simulink model "RadarSimulinkProjectRev001b"  (R2024a)
settings: Solver=VariableStepAuto  StartTime=0.0  StopTime=0.001  RelTol=1e-3
values from neighbouring files (symbols this model uses):
  AngleTime = SweepTime/10    (= 10000)    [InitializationOfVariables.m]    (also in InitializationOfVariablesRev000.m; InitializationOfVariablesRev001.m; InitializationOfVariablesRev003.m = 2097152; InitializationOfVariablesRev004.m = 2097152)
  Btn_Debounce = 20000    [InitializationOfVariablesRev003.m]    (also in InitializationOfVariablesRev004.m)
  FreqDeltaPeriod = 45    [InitializationOfVariablesRev003.m]    (also in InitializationOfVariablesRev004.m = 1)
  RXFFTLength = 16384    [InitializationOfVariablesRev003.m]    (also in InitializationOfVariablesRev004.m = 2048)
  SweepTime = 100000    [InitializationOfVariables.m]    (also in InitializationOfVariablesRev000.m; InitializationOfVariablesRev001.m; InitializationOfVariablesRev003.m = 23068672; InitializationOfVariablesRev004.m = 23068672)
undefined symbols (not defined in the file or in its folder): SignalGenerationForAnalysis, Subsystem, xc7a200tfbg676
libraries: hdlBasic x75, hdlDSPIP x6, hdlUtilities x1, vmcUtilities x1
settings Model: Creator=Cube II  LastModifiedBy=Cube II

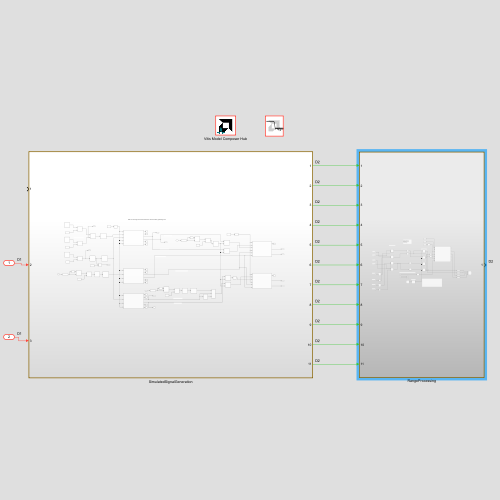
[thumbnail: Simulink's stored preview of the top-level diagram]
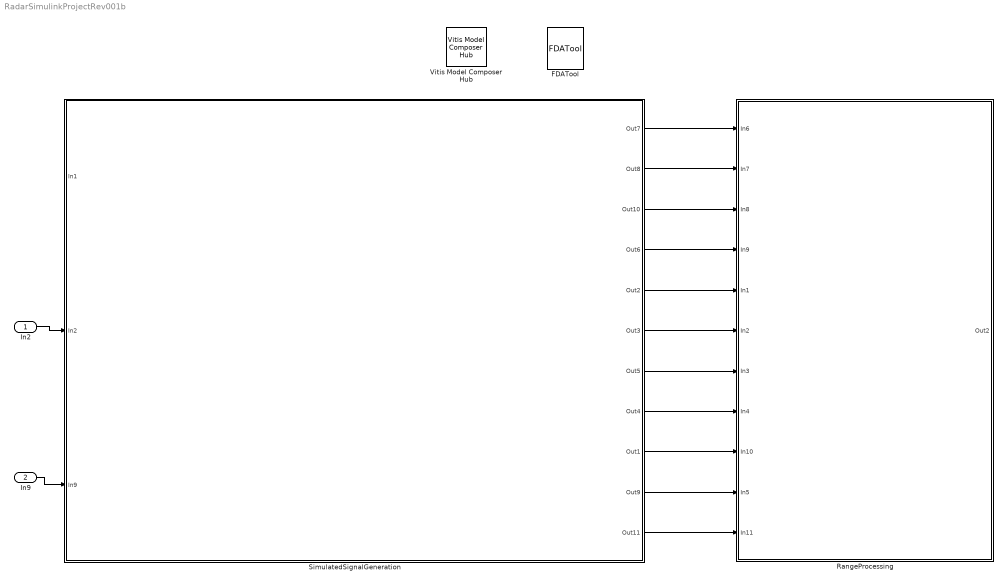
== system RadarSimulinkProjectRev001b ==
  In2 : Inport
  In9 : Inport  Port=2
  FDATool : hdlUtilities/FDATool  block_type=fdatool
      settings: infoedit=FDATool
  RangeProcessing : Subsystem
  SimulatedSignalGeneration : Subsystem  SystemSampleTime=1/200e6
  Vitis Model Composer Hub : vmcUtilities/Vitis Model Composer Hub  Tag=genX  CodeGeneration=off  SubsystemName=Subsystem  BlockHierPath=SignalGenerationForAnalysis/Subsystem  CompilationType=HDLCompilation  SubsystemType=HDLNode  ExportTypeV2=IP Catalog  StartColumn=1  NumberOfColumns=1  TargetDirectory=./netlist  exportDesign=off  analyzeDesign=on  validateDesignOnHw=off  ExportType=AI Engines  IpVendor=xilinx.com  IpLibrary=hls  IpVersion=1.0  IpHWLanguage=Verilog  AieCompilerOptions={}  AieSimulatorOptions={}  CreateTestbench=on  TestbenchStackSize=10  RunRtlSim=off  RunCSim=off  RunAieSim=off  AieSimTimeout=50000  RunAieSimProfiling=off  LaunchVitisAnalyzer=off  PlotOutput=off  RunX86Sim=off  X86SimTimeout=10  GenHwImage=off  GenLibadfXo=on  GenHwValidationCode=off  PlatformType=Not Specified  HwSystemType=Baremetal  HwValidationTarget=hw  ProjDevice=Artix-7 AC701 Evaluation Platform (xc7a200tfbg676-2)  ProjDevicePart=xc7a200tfbg676-2  AIEType=None  SamplePeriod=-1  ClockFrequency=200  DataPathParallelism=1  xilinxfamily=artix7  part=xc7a200t  speed=-2  package=fbg676  directory=./netlist\ip\Subsystem\src  testbench=off  incr_netlist=off  synthesis_tool=Vivado  clock_wrapper=Clock Enables  dbl_ovrd=According to Block Masks  dcm_input_clock_period=10  sysclk_period=5  simulink_period=1/200e6  eval_field=0  IPInfoJsonString="{\"DUTSubsystemName\":\"Subsystem\",\"HDLSubsystem\":{\"SubsystemName\":\"Subsystem\",\"IPName\":\"Subsystem\",\"IPLibrary\":\"VMC\",\"IPVendor\":\"User Company\",\"IPVersion\":\"1.0\",\"TargetDirectory\":\"./netlist\",\"SubsystemDir\":\"./netlist\\\\ip\\\\Subsystem\",\"FreqHz\":\"200000000\"},\"SubsystemTag\":\"HDLNode\"}"  LogFileName=S:\RadarProjectSimulink\netlist\model_composer.log  NThreads=4  IPConfigFile=C:\Users\Cube II\AppData\Local\Temp\vmctmp-5941030035629153029\SignalGenerationForAnalysis_ipconfig.json
  wires:
  In2/1 -> SimulatedSignalGeneration/2(In2)
  In9/1 -> SimulatedSignalGeneration/3(In9)
  SimulatedSignalGeneration/3(Out10) -> RangeProcessing/3(In8)
  SimulatedSignalGeneration/4(Out6) -> RangeProcessing/4(In9)
  SimulatedSignalGeneration/7(Out5) -> RangeProcessing/7(In3)
  SimulatedSignalGeneration/8(Out4) -> RangeProcessing/8(In4)
  SimulatedSignalGeneration/10(Out9) -> RangeProcessing/10(In5)
  SimulatedSignalGeneration/9(Out1) -> RangeProcessing/9(In10)
  SimulatedSignalGeneration/2(Out8) -> RangeProcessing/2(In7)
  SimulatedSignalGeneration/1(Out7) -> RangeProcessing/1(In6)
  SimulatedSignalGeneration/6(Out3) -> RangeProcessing/6(In2)
  SimulatedSignalGeneration/5(Out2) -> RangeProcessing/5(In1)
  SimulatedSignalGeneration/11(Out11) -> RangeProcessing/11(In11)

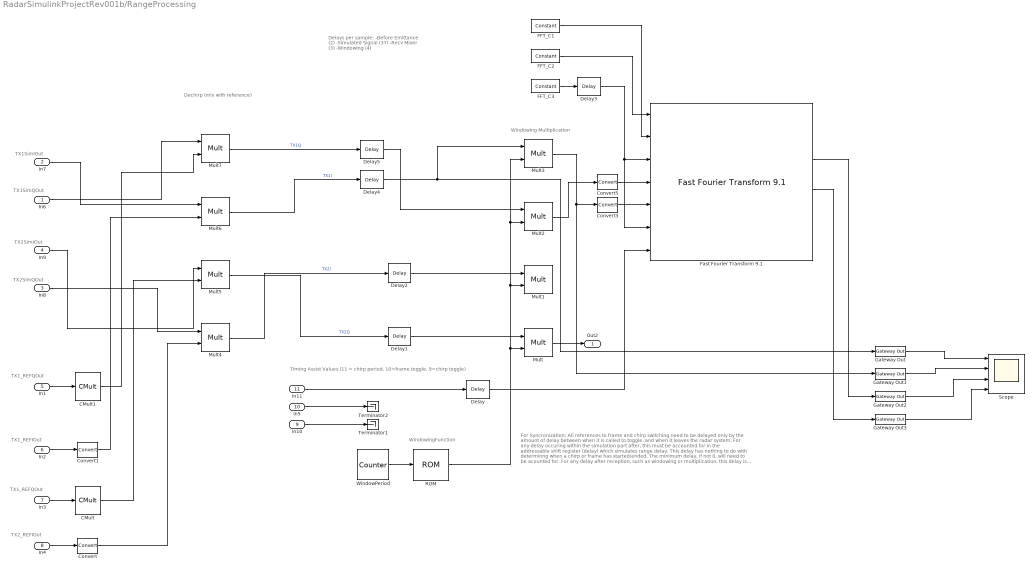
== system RadarSimulinkProjectRev001b/RangeProcessing ==
  note: Delays per sample:
      | -Before Emittance (2)
      | -Simulated Signal (37)
      | -Recv Mixer (3)
      | -Windowing (4)
  note: TX1SimIOut
  note: TX1SimQOut
  note: TX2SimIOut
  note: TX2SimQOut
  note: TX1_REFIOut
  note: TX1_REFQOut
  note: TX2_REFIOut
  note: TX1_REFQOut
  note: Dechirp (mix with reference)
  note: Timing Assist Values (11 = chirp period, 10=frame toggle, 9=chirp toggle)
  note: WindowingFunction
  note: Windowing Multiplication
  note: For Syncronization: All references to frame and chirp switching need to be delayed only by the amount of delay between when it is called to toggle, and when it leaves the radar system.
      |
      | For any delay occuring within the simulation part after, this must be accounted for in the addressable shift register (delay) which simulates range delay. This delay has nothing to do with determinng when a chirp or frame has started/ended. The minimum delay, if not 0, will need to be acounted for.
      |
      | For any delay after reception, such as windowing or multiplication, this delay is relevant to anything that has to do with the processes that depend on knowing when a frame or chirp has started/ended. Since it should only start sampling once a signal theoretically should have arrived from 0 meters (no sim delay)
  In6 : Inport
  In7 : Inport  Port=2
  In8 : Inport  Port=3
  In9 : Inport  Port=4
  In1 : Inport  Port=5
  In2 : Inport  Port=6
  In3 : Inport  Port=7
  In4 : Inport  Port=8
  In10 : Inport  Port=9
  In5 : Inport  Port=10
  In11 : Inport  Port=11
  CMult : hdlBasic/CMult  const=-1  gui_display_data_type=Fixed-point  const_n_bits=1  const_bin_pt=0  float_type=Single  exp_bits=8  fraction_bits=24  en=off  latency=0  precision=Full  arith_type="Signed  (2's comp)"  n_bits=16  bin_pt=14  quantization=Truncate  overflow=Wrap  use_behavioral_HDL=off  mem_type=Distributed RAM  pipeline=off  XmcBlockStatus=1  maskContainerNames=tabcontainer1  block_type=cmult  block_config=sysgen:CMult_config
      settings: infoedit=[]
  CMult1 : hdlBasic/CMult  const=-1  gui_display_data_type=Fixed-point  const_n_bits=1  const_bin_pt=0  float_type=Single  exp_bits=8  fraction_bits=24  en=off  latency=0  precision=Full  arith_type="Signed  (2's comp)"  n_bits=16  bin_pt=14  quantization=Truncate  overflow=Wrap  use_behavioral_HDL=off  mem_type=Distributed RAM  pipeline=off  XmcBlockStatus=1  maskContainerNames=tabcontainer1  block_type=cmult  block_config=sysgen:CMult_config
      settings: infoedit=[]
  Convert : hdlBasic/Convert  gui_display_data_type=Fixed-point  arith_type=Signed (2's comp)  n_bits=17  bin_pt=15  float_type=Single  exp_bits=8  fraction_bits=24  quantization=Truncate  overflow=Wrap  en=off  latency=0  pipeline=off  XmcBlockStatus=1  maskContainerNames=group2  block_type=convert  block_config=sysgen:Convert_config  block_width=595  block_height=885
  Convert1 : hdlBasic/Convert  gui_display_data_type=Fixed-point  arith_type=Signed (2's comp)  n_bits=17  bin_pt=15  float_type=Single  exp_bits=8  fraction_bits=24  quantization=Truncate  overflow=Wrap  en=off  latency=0  pipeline=off  XmcBlockStatus=1  maskContainerNames=group2  block_type=convert  block_config=sysgen:Convert_config  block_width=595  block_height=885
  Convert3 : hdlBasic/Convert  gui_display_data_type=Fixed-point  arith_type=Signed (2's comp)  n_bits=16  bin_pt=15  float_type=Single  exp_bits=8  fraction_bits=24  quantization=Truncate  overflow=Wrap  en=off  latency=0  pipeline=off  XmcBlockStatus=1  maskContainerNames=group2  block_type=convert  block_config=sysgen:Convert_config  block_width=595  block_height=885
  Convert5 : hdlBasic/Convert  gui_display_data_type=Fixed-point  arith_type=Signed (2's comp)  n_bits=16  bin_pt=15  float_type=Single  exp_bits=8  fraction_bits=24  quantization=Truncate  overflow=Wrap  en=off  latency=0  pipeline=off  XmcBlockStatus=1  maskContainerNames=group2  block_type=convert  block_config=sysgen:Convert_config  block_width=595  block_height=885
  Delay : hdlBasic/Delay  rst=off  en=off  latency=46  reg_retiming=off  XmcBlockStatus=1  maskContainerNames=group1  block_type=delay  block_config=sysgen:Delay_config
  Delay{1..2,4..5} (4 alike) : hdlBasic/Delay  rst=off  en=off  latency=1  reg_retiming=off  XmcBlockStatus=1  maskContainerNames=group1  block_type=delay  block_config=sysgen:Delay_config
  Delay3 : hdlBasic/Delay  rst=off  en=off  latency=46  reg_retiming=off  XmcBlockStatus=1  maskContainerNames=group1  block_type=delay  block_config=sysgen:Delay_config
  FFT_C1 : hdlBasic/Constant  const=1.0  gui_display_data_type=Fixed-point  arith_type=Unsigned  n_bits=1  bin_pt=0  preci_type=Single  exp_width=8  frac_width=24  explicit_period=on  period=1/200e6  XmcBlockStatus=1  maskContainerNames=tabcontainer1  block_type=constant  block_config=sysgen:Constant_config
  FFT_C2 : hdlBasic/Constant  const=0  gui_display_data_type=Fixed-point  arith_type=Unsigned  n_bits=12  bin_pt=0  preci_type=Single  exp_width=8  frac_width=24  explicit_period=on  period=1/200e6  XmcBlockStatus=1  maskContainerNames=tabcontainer1  block_type=constant  block_config=sysgen:Constant_config
  FFT_C3 : hdlBasic/Constant  const=1  gui_display_data_type=Boolean  arith_type=Boolean  n_bits=12  bin_pt=0  preci_type=Single  exp_width=8  frac_width=24  explicit_period=on  period=1/200e6  XmcBlockStatus=1  maskContainerNames=tabcontainer1  block_type=constant  block_config=sysgen:Constant_config
  Fast Fourier Transform 9.1 : hdlDSPIP/Fast Fourier Transform 9.1   transform_length=4096  target_clock_frequency=200  target_data_throughput=50  implementation_options=pipelined_streaming_io  run_time_configurable_transform_length=off  enable_ssr=off  super_sample_rates=1  data_format=fixed_point  phase_factor_width=24  scaling_options=scaled  rounding_modes=truncation  aclken=off  aresetn=off  output_ordering=bit_reversed_order  cyclic_prefix_insertion=off  throttle_scheme=realtime  xk_index=off  ovflo=off  trim_axipin_name=on  memory_options_data=block_ram  memory_options_phase_factors=block_ram  number_of_stages_using_block_ram_for_data_and_phase_factors=4  memory_options_reorder=block_ram  memory_options_hybrid=off  complex_mult_type=use_mults_resources  butterfly_type=use_luts  simulation_type=hybrid_sim  simulation_model=sysgen:xfftv9_cmodel  data_path_portlist={ 's_axis_data_tdata', 'm_axis_data_tdata', 'm_axis_status_tdata', 'event_fft_overflow' }  channels=1  input_ordering=natural_order  input_width=16  ip_name=Fast Fourier Transform  ip_version=9.1  dsptool_ready=true  ipcore_usecache=true  ipcore_useipmodelcache=true  wrapper_available=true  port_translation_map={ 'aclken' => 'en', 'aresetn' => 'rst'}  XmcBlockStatus=1  maskContainerNames=tabcontainer1  block_type=xfft_v9_1  block_config=sysgen:rodinimport_config
  Gateway Out{,1..3} (4 alike) : hdlBasic/Gateway Out  inherit_from_input=off  bool_to_boolean=off  hdl_port=on  rows=1  columns=1  UseAsDAC=off  DACChannel='1'  interface=None  automatic_assignment=on  address_offset=hex2dec('00')  intf_name=''  intf_description=''  timing_constraint=None  locs_specified=off  LOCs={}  io_standard={}  XmcBlockStatus=1  maskContainerNames=group4  block_type=gatewayout  block_config=sysgen:gateway_out_config  block_width_w=590  block_height_w=620  block_width=620  block_height=750
  Mult{,1..7} (8 alike) : hdlBasic/Mult  precision=Full  arith_type="Signed  (2's comp)"  n_bits=16  bin_pt=14  quantization=Truncate  overflow=Wrap  en=off  latency=3  opt_float=off  fp_mult_usage=No Usage  use_behavioral_HDL=off  opt=Speed  use_embedded=on  optimum_pipeline=off  pipeline=on  use_rpm=on  placement_style=Triangular  XmcBlockStatus=1  maskContainerNames=group1  block_type=mult  block_config=sysgen:Mult_config  block_width=598  block_height=876
  ROM : hdlBasic/ROM  depth=RXFFTLength  initVector=WindowCoefficients  distributed_mem=Block RAM  rst=off  init_reg=0  en=off  latency=1  gui_display_data_type=Fixed-point  arith_type=Unsigned  n_bits=16  bin_pt=16  preci_type=Single  exp_width=8  frac_width=24  optimize=Area  use_rpm=on  simulation_type=fast_sim  XmcBlockStatus=1  maskContainerNames=tabcontainer1  block_type=sprom  block_config=sysgen:SPROM_config
  Scope : Scope  NumInputPorts=4
  Terminator1 : Terminator
  Terminator2 : Terminator
  WindowPeriod : hdlBasic/Counter  cnt_type=Count limited  cnt_to=RXFFTLength-1  operation=Up  start_count=0  cnt_by_val=1  arith_type=Unsigned  n_bits=12  bin_pt=0  load_pin=off  rst=off  en=off  explicit_period=Explicit  period=1/200e6  use_behavioral_HDL=off  implementation=Fabric  XmcBlockStatus=1  maskContainerNames=group1  block_type=counter  block_config=sysgen:Counter_config  block_width=531  block_height=1023
  Out2 : Outport
  wires:
  ROM/1 -> Mult3/2, Mult2/2, Mult1/2, Mult/2
  Mult/1 -> Out2/1
  WindowPeriod/1 -> ROM/1
  In4/1 -> Convert/1
  In3/1 -> CMult/1
  In2/1 -> Convert1/1
  In1/1 -> CMult1/1
  In10/1 -> Terminator1/1
  Mult2/1 -> Convert5/1
  Mult3/1 -> Convert3/1, Gateway Out1/1
  FFT_C1/1 -> Fast Fourier Transform 9.1/2
  FFT_C2/1 -> Fast Fourier Transform 9.1/1
  FFT_C3/1 -> Delay3/1
  Convert3/1 -> Fast Fourier Transform 9.1/5
  Convert5/1 -> Fast Fourier Transform 9.1/4
  Delay3/1 -> Fast Fourier Transform 9.1/3, Fast Fourier Transform 9.1/6
  Gateway Out/1 -> Scope/1
  Gateway Out1/1 -> Scope/2
  Gateway Out2/1 -> Scope/3
  Fast Fourier Transform 9.1/4 -> Gateway Out2/1
  In7/1 -> Mult6/1
  In6/1 -> Mult7/1
  CMult1/1 -> Mult7/2
  Convert1/1 -> Mult6/2
  In9/1 -> Mult5/1
  In8/1 -> Mult4/1
  CMult/1 -> Mult5/2
  Convert/1 -> Mult4/2
  Mult5/1 -> Delay1/1  "TX2Q"
  Mult4/1 -> Delay2/1  "TX2I"
  Mult6/1 -> Delay4/1  "TX1I"
  Mult7/1 -> Delay5/1  "TX1Q"
  Delay1/1 -> Mult/1
  Delay2/1 -> Mult1/1
  Delay4/1 -> Mult3/1, Gateway Out/1
  Delay5/1 -> Mult2/1
  Gateway Out3/1 -> Scope/4
  Fast Fourier Transform 9.1/6 -> Gateway Out3/1
  In11/1 -> Delay/1
  Delay/1 -> Fast Fourier Transform 9.1/7
  In5/1 -> Terminator2/1

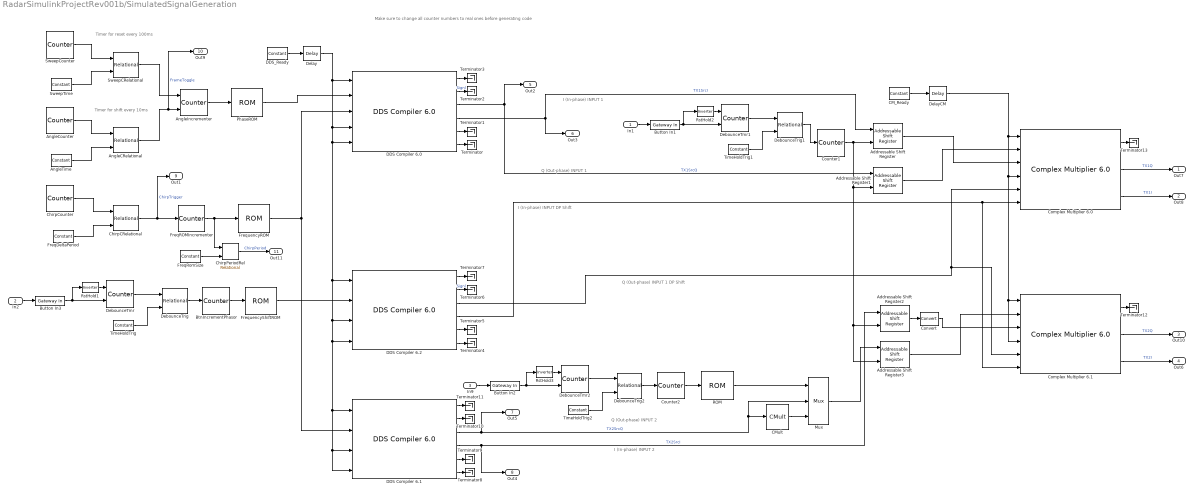
== system RadarSimulinkProjectRev001b/SimulatedSignalGeneration ==
  note: Make sure to change all counter numbers to real ones before generating code
  note: Timer for shift every 10ms
  note: Timer for reset every 100ms
  note: I (In-phase) INPUT 1
  note: Q (Out-phase) INPUT 1
  note: Q (Out-phase) INPUT 2
  note: Q (Out-phase) INPUT 1 DP Shift
  note: I (In-phase) INPUT DP Shift
  note: I (In-phase) INPUT 2
  In1 : Inport
  In2 : Inport  Port=2
  In9 : Inport  Port=3
  Addressable Shift Register{,1..3} (4 alike) : hdlBasic/Addressable Shift Register  infer_latency=off  depth=10  initVector=ASR_LUT  en=off  use_behavioral_HDL=off  Optimization=Resource  XmcBlockStatus=1  maskContainerNames=group1  block_type=addrsr  block_config=sysgen:Addrsr_config
  AngleCRelational : hdlBasic/Relational  mode=a=b  op_type=Bool  en=off  latency=0  XmcBlockStatus=1  maskContainerNames=tabcontainer1  block_type=relational  block_config=sysgen:Relational_config
  AngleCounter : hdlBasic/Counter  cnt_type=Count limited  cnt_to=AngleTime-1  operation=Up  start_count=0  cnt_by_val=1  arith_type=Unsigned  n_bits=32  bin_pt=0  load_pin=off  rst=off  en=off  explicit_period=Explicit  period=1/200e6  use_behavioral_HDL=off  implementation=Fabric  XmcBlockStatus=1  maskContainerNames=group1  block_type=counter  block_config=sysgen:Counter_config  block_width=531  block_height=1023
  AngleIncrementer : hdlBasic/Counter  cnt_type=Count limited  cnt_to=10  operation=Up  start_count=0  cnt_by_val=1  arith_type=Unsigned  n_bits=4  bin_pt=0  load_pin=off  rst=on  en=on  explicit_period=Inferred from inputs  period=1/100  use_behavioral_HDL=off  implementation=Fabric  XmcBlockStatus=1  maskContainerNames=group1  block_type=counter  block_config=sysgen:Counter_config  block_width=531  block_height=1023
  AngleTime : hdlBasic/Constant  const=AngleTime-1  gui_display_data_type=Fixed-point  arith_type=Unsigned  n_bits=24  bin_pt=0  preci_type=Single  exp_width=8  frac_width=24  explicit_period=off  period=1  XmcBlockStatus=1  maskContainerNames=tabcontainer1  block_type=constant  block_config=sysgen:Constant_config
  BtnIncrementPhasor : hdlBasic/Counter  cnt_type=Count limited  cnt_to=8  operation=Up  start_count=0  cnt_by_val=1  arith_type=Unsigned  n_bits=4  bin_pt=0  load_pin=off  rst=off  en=on  explicit_period=Explicit  period=1/200e6  use_behavioral_HDL=off  implementation=Fabric  XmcBlockStatus=1  maskContainerNames=group1  block_type=counter  block_config=sysgen:Counter_config  block_width=531  block_height=1023
  Button In1 : hdlBasic/Gateway In  gui_display_data_type=Boolean  arith_type=Boolean  n_bits=16  bin_pt=14  preci_type=Single  exp_width=8  frac_width=24  rows=1  columns=1  quantization="Round  (unbiased: +/- Inf)"  overflow=Saturate  period=1/200e6  UseAsADC=off  ADCChannel='1'  interface=None  automatic_assignment=on  address_offset=hex2dec('00')  intf_name=''  intf_description=''  default_value=0  timing_constraint=None  locs_specified=off  LOCs={}  io_standard={}  inherit_from_input=off  hdl_port=on  XmcBlockStatus=1  maskContainerNames=group4  block_type=gatewayin  block_config=sysgen:gateway_in_config  block_width_w=590  block_height_w=620  block_width=640  block_height=850
  Button In2 : hdlBasic/Gateway In  gui_display_data_type=Boolean  arith_type=Boolean  n_bits=16  bin_pt=14  preci_type=Single  exp_width=8  frac_width=24  rows=1  columns=1  quantization="Round  (unbiased: +/- Inf)"  overflow=Saturate  period=1/200e6  UseAsADC=off  ADCChannel='1'  interface=None  automatic_assignment=on  address_offset=hex2dec('00')  intf_name=''  intf_description=''  default_value=0  timing_constraint=None  locs_specified=off  LOCs={}  io_standard={}  inherit_from_input=off  hdl_port=on  XmcBlockStatus=1  maskContainerNames=group4  block_type=gatewayin  block_config=sysgen:gateway_in_config  block_width_w=590  block_height_w=620  block_width=640  block_height=850
  Button In3 : hdlBasic/Gateway In  gui_display_data_type=Boolean  arith_type=Boolean  n_bits=16  bin_pt=14  preci_type=Single  exp_width=8  frac_width=24  rows=1  columns=1  quantization="Round  (unbiased: +/- Inf)"  overflow=Saturate  period=1/200e6  UseAsADC=off  ADCChannel='1'  interface=None  automatic_assignment=on  address_offset=hex2dec('00')  intf_name=''  intf_description=''  default_value=0  timing_constraint=None  locs_specified=off  LOCs={}  io_standard={}  inherit_from_input=off  hdl_port=on  XmcBlockStatus=1  maskContainerNames=group4  block_type=gatewayin  block_config=sysgen:gateway_in_config  block_width_w=590  block_height_w=620  block_width=640  block_height=850
  CM_Ready : hdlBasic/Constant  const=1  gui_display_data_type=Boolean  arith_type=Boolean  n_bits=24  bin_pt=0  preci_type=Single  exp_width=8  frac_width=24  explicit_period=on  period=1/200e6  XmcBlockStatus=1  maskContainerNames=tabcontainer1  block_type=constant  block_config=sysgen:Constant_config
  CMult : hdlBasic/CMult  const=-1  gui_display_data_type=Fixed-point  const_n_bits=1  const_bin_pt=0  float_type=Single  exp_bits=8  fraction_bits=24  en=off  latency=0  precision=Full  arith_type="Signed  (2's comp)"  n_bits=16  bin_pt=14  quantization=Truncate  overflow=Wrap  use_behavioral_HDL=off  mem_type=Distributed RAM  pipeline=off  XmcBlockStatus=1  maskContainerNames=tabcontainer1  block_type=cmult  block_config=sysgen:CMult_config
      settings: infoedit=[]
  ChirpCRelational : hdlBasic/Relational  mode=a=b  op_type=Bool  en=off  latency=0  XmcBlockStatus=1  maskContainerNames=tabcontainer1  block_type=relational  block_config=sysgen:Relational_config
  ChirpCounter : hdlBasic/Counter  cnt_type=Count limited  cnt_to=FreqDeltaPeriod  operation=Up  start_count=0  cnt_by_val=1  arith_type=Unsigned  n_bits=8  bin_pt=0  load_pin=off  rst=off  en=off  explicit_period=Explicit  period=1/200e6  use_behavioral_HDL=off  implementation=Fabric  XmcBlockStatus=1  maskContainerNames=group1  block_type=counter  block_config=sysgen:Counter_config  block_width=531  block_height=1023
  ChirpPeriodRel : hdlBasic/Relational  mode=a=b  op_type=Bool  en=off  latency=0  XmcBlockStatus=1  maskContainerNames=tabcontainer1  block_type=relational  block_config=sysgen:Relational_config
  Complex Multiplier 6.0 : hdlDSPIP/Complex Multiplier 6.0   datatype=integer  hasatlast=off  hasatuser=off  atuserwidth=1  hasbtlast=off  hasbtuser=off  btuserwidth=1  multtype=Use_Mults  optimizegoal=Resources  flowcontrol=NonBlocking  outputwidth=34  roundmode=Truncate  hasctrltlast=off  hasctrltuser=off  ctrltuserwidth=1  outtlastbehv=Null  latencyconfig=Automatic  minimumlatency=37  aclken=off  aresetn=off  trim_axipin_name=on  simulation_type=hybrid_sim  simulation_model=sysgen:cmpy_v6_0  data_path_portlist={ 's_axis_a_tdata_real', 's_axis_a_tdata_imag', 's_axis_b_tdata_real', 's_axis_b_tdata_imag', 's_axis_ctrl_tdata_rounding_bit', 'm_axis_dout_tdata_real', 'm_axis_dout_tdata_imag' }  aportwidth=63  bportwidth=63  ip_name=Complex Multiplier  ip_version=6.0  dsptool_ready=true  ipcore_usecache=true  ipcore_useipmodelcache=true  ipcore_verbose=false  ipcore_latency_parameter='minimumlatency'  wrapper_available=true  port_translation_map={ 'aclken' => 'en', 'aresetn' => 'rst'}  XmcBlockStatus=1  maskContainerNames=tabcontainer1  block_type=cmpy_v6_0  block_config=sysgen:rodinimport_config
  Complex Multiplier 6.1 : hdlDSPIP/Complex Multiplier 6.0   datatype=integer  hasatlast=off  hasatuser=off  atuserwidth=1  hasbtlast=off  hasbtuser=off  btuserwidth=1  multtype=Use_Mults  optimizegoal=Resources  flowcontrol=NonBlocking  outputwidth=34  roundmode=Truncate  hasctrltlast=off  hasctrltuser=off  ctrltuserwidth=1  outtlastbehv=Null  latencyconfig=Automatic  minimumlatency=37  aclken=off  aresetn=off  trim_axipin_name=on  simulation_type=hybrid_sim  simulation_model=sysgen:cmpy_v6_0  data_path_portlist={ 's_axis_a_tdata_real', 's_axis_a_tdata_imag', 's_axis_b_tdata_real', 's_axis_b_tdata_imag', 's_axis_ctrl_tdata_rounding_bit', 'm_axis_dout_tdata_real', 'm_axis_dout_tdata_imag' }  aportwidth=63  bportwidth=63  ip_name=Complex Multiplier  ip_version=6.0  dsptool_ready=true  ipcore_usecache=true  ipcore_useipmodelcache=true  ipcore_verbose=false  ipcore_latency_parameter='minimumlatency'  wrapper_available=true  port_translation_map={ 'aclken' => 'en', 'aresetn' => 'rst'}  XmcBlockStatus=1  maskContainerNames=tabcontainer1  block_type=cmpy_v6_0  block_config=sysgen:rodinimport_config
  Convert : hdlBasic/Convert  gui_display_data_type=Fixed-point  arith_type=Signed (2's comp)  n_bits=17  bin_pt=15  float_type=Single  exp_bits=8  fraction_bits=24  quantization=Truncate  overflow=Wrap  en=off  latency=0  pipeline=off  XmcBlockStatus=1  maskContainerNames=group2  block_type=convert  block_config=sysgen:Convert_config  block_width=595  block_height=885
  Counter1 : hdlBasic/Counter  cnt_type=Count limited  cnt_to=9  operation=Up  start_count=0  cnt_by_val=1  arith_type=Unsigned  n_bits=4  bin_pt=0  load_pin=off  rst=off  en=on  explicit_period=Explicit  period=1/200e6  use_behavioral_HDL=off  implementation=Fabric  XmcBlockStatus=1  maskContainerNames=group1  block_type=counter  block_config=sysgen:Counter_config  block_width=531  block_height=1023
  Counter2 : hdlBasic/Counter  cnt_type=Count limited  cnt_to=1  operation=Up  start_count=0  cnt_by_val=1  arith_type=Unsigned  n_bits=1  bin_pt=0  load_pin=off  rst=off  en=on  explicit_period=Explicit  period=1/200e6  use_behavioral_HDL=off  implementation=Fabric  XmcBlockStatus=1  maskContainerNames=group1  block_type=counter  block_config=sysgen:Counter_config  block_width=531  block_height=1023
  DDS Compiler 6.0 : hdlDSPIP/DDS Compiler 6.0   partspresent=Phase_Generator_and_SIN_COS_LUT  dds_clock_rate=200  channels=1  mode_of_operation=Standard  output_type=Integer  modulus=9  parameter_entry=Hardware_Parameters  spurious_free_dynamic_range=45  frequency_resolution=0.4  noise_shaping=None  phase_width=24  output_width=16  output_selection=Sine_and_Cosine  negative_sine=off  negative_cosine=off  amplitude_mode=Full_Range  memory_type=Auto  optimization_goal=Auto  dsp48_use=Minimal  resync=off  latency_configuration=Auto  latency=1  has_phase_out=on  has_aclken=off  has_aresetn=off  explicit_period=on  period=1/200e6  data_has_tlast=Not_Required  has_tready=on  s_phase_has_tuser=Not_Required  m_data_has_tuser=Not_Required  m_phase_has_tuser=Not_Required  s_phase_tuser_width=1  output_form=Twos_Complement  s_config_sync_mode=On_Vector  phase_increment=Streaming  output_frequency1=0  output_frequency2=0  output_frequency3=0  output_frequency4=0  output_frequency5=0  output_frequency6=0  output_frequency7=0  output_frequency8=0  output_frequency9=0  output_frequency10=0  output_frequency11=0  output_frequency12=0  output_frequency13=0  output_frequency14=0  output_frequency15=0  output_frequency16=0  pinc1='0'  pinc2='0'  pinc3='0'  pinc4='0'  pinc5='0'  pinc6='0'  pinc7='0'  pinc8='0'  pinc9='0'  pinc10='0'  pinc11='0'  pinc12='0'  pinc13='0'  pinc14='0'  pinc15='0'  pinc16='0'  phase_offset=Streaming  phase_offset_angles1=0  phase_offset_angles2=0  phase_offset_angles3=0  phase_offset_angles4=0  phase_offset_angles5=0  phase_offset_angles6=0  phase_offset_angles7=0  phase_offset_angles8=0  phase_offset_angles9=0  phase_offset_angles10=0  phase_offset_angles11=0  phase_offset_angles12=0  phase_offset_angles13=0  phase_offset_angles14=0  phase_offset_angles15=0  phase_offset_angles16=0  poff1='0'  poff2='0'  poff3='0'  poff4='0'  poff5='0'  poff6='0'  poff7='0'  poff8='0'  poff9='0'  poff10='0'  poff11='0'  poff12='0'  poff13='0'  poff14='0'  poff15='0'  poff16='0'  trim_axipin_name=on  simulation_type=hybrid_sim  simulation_model=sysgen:xddsv6_0_cmodel  data_path_portlist={ 's_axis_config_tdata_poff', 's_axis_config_tdata_chan0_poff', 's_axis_config_tdata_pinc', 's_axis_config_tdata_chan0_pinc', 's_axis_phase_tdata_resync', 's_axis_phase_tdata_chan0_resync', 's_axis_phase_tdata_poff', 's_axis_phase_tdata_chan0_poff', 's_axis_phase_tdata_pinc', 's_axis_phase_tdata_chan0_pinc', 's_axis_phase_tdata_phase_in', 'm_axis_data_tdata_sine', 'm_axis_data_tdata_chan0_sine', 'm_axis_data_tdata_cosine', 'm_axis_data_tdata_chan0_cosine', 'm_axis_phase_tdata_phase_out', 'm_axis_phase_tdata_chan0_phase_out'}  por_mode=false  gui_behaviour=Sysgen  ip_name=DDS Compiler  ip_version=6.0  dsptool_ready=true  wrapper_available=true  port_translation_map={ 'aclken' => 'en', 'aresetn' => 'rst' }  ipcore_usecache=true  ipcore_useipmodelcache=true  ipcore_xco_need_fpga_part=true  ipcore_fpga_part=[]  ipcore_verbose=false  XmcBlockStatus=1  maskContainerNames=tabcontainer1  block_type=dds_compiler_v6_0  block_config=sysgen:rodinimport_config  block_width=760
  DDS Compiler 6.1 : hdlDSPIP/DDS Compiler 6.0   partspresent=Phase_Generator_and_SIN_COS_LUT  dds_clock_rate=200  channels=1  mode_of_operation=Standard  output_type=Integer  modulus=9  parameter_entry=Hardware_Parameters  spurious_free_dynamic_range=45  frequency_resolution=0.4  noise_shaping=None  phase_width=24  output_width=16  output_selection=Sine_and_Cosine  negative_sine=off  negative_cosine=off  amplitude_mode=Full_Range  memory_type=Auto  optimization_goal=Auto  dsp48_use=Minimal  resync=off  latency_configuration=Auto  latency=1  has_phase_out=on  has_aclken=off  has_aresetn=off  explicit_period=on  period=1/200e6  data_has_tlast=Not_Required  has_tready=on  s_phase_has_tuser=Not_Required  m_data_has_tuser=Not_Required  m_phase_has_tuser=Not_Required  s_phase_tuser_width=1  output_form=Twos_Complement  s_config_sync_mode=On_Vector  phase_increment=Streaming  output_frequency1=0  output_frequency2=0  output_frequency3=0  output_frequency4=0  output_frequency5=0  output_frequency6=0  output_frequency7=0  output_frequency8=0  output_frequency9=0  output_frequency10=0  output_frequency11=0  output_frequency12=0  output_frequency13=0  output_frequency14=0  output_frequency15=0  output_frequency16=0  pinc1='0'  pinc2='0'  pinc3='0'  pinc4='0'  pinc5='0'  pinc6='0'  pinc7='0'  pinc8='0'  pinc9='0'  pinc10='0'  pinc11='0'  pinc12='0'  pinc13='0'  pinc14='0'  pinc15='0'  pinc16='0'  phase_offset=Fixed  phase_offset_angles1=0  phase_offset_angles2=0  phase_offset_angles3=0  phase_offset_angles4=0  phase_offset_angles5=0  phase_offset_angles6=0  phase_offset_angles7=0  phase_offset_angles8=0  phase_offset_angles9=0  phase_offset_angles10=0  phase_offset_angles11=0  phase_offset_angles12=0  phase_offset_angles13=0  phase_offset_angles14=0  phase_offset_angles15=0  phase_offset_angles16=0  poff1='0'  poff2='0'  poff3='0'  poff4='0'  poff5='0'  poff6='0'  poff7='0'  poff8='0'  poff9='0'  poff10='0'  poff11='0'  poff12='0'  poff13='0'  poff14='0'  poff15='0'  poff16='0'  trim_axipin_name=on  simulation_type=hybrid_sim  simulation_model=sysgen:xddsv6_0_cmodel  data_path_portlist={ 's_axis_config_tdata_poff', 's_axis_config_tdata_chan0_poff', 's_axis_config_tdata_pinc', 's_axis_config_tdata_chan0_pinc', 's_axis_phase_tdata_resync', 's_axis_phase_tdata_chan0_resync', 's_axis_phase_tdata_poff', 's_axis_phase_tdata_chan0_poff', 's_axis_phase_tdata_pinc', 's_axis_phase_tdata_chan0_pinc', 's_axis_phase_tdata_phase_in', 'm_axis_data_tdata_sine', 'm_axis_data_tdata_chan0_sine', 'm_axis_data_tdata_cosine', 'm_axis_data_tdata_chan0_cosine', 'm_axis_phase_tdata_phase_out', 'm_axis_phase_tdata_chan0_phase_out'}  por_mode=false  gui_behaviour=Sysgen  ip_name=DDS Compiler  ip_version=6.0  dsptool_ready=true  wrapper_available=true  port_translation_map={ 'aclken' => 'en', 'aresetn' => 'rst' }  ipcore_usecache=true  ipcore_useipmodelcache=true  ipcore_xco_need_fpga_part=true  ipcore_fpga_part=[]  ipcore_verbose=false  XmcBlockStatus=1  maskContainerNames=tabcontainer1  block_type=dds_compiler_v6_0  block_config=sysgen:rodinimport_config  block_width=760
  DDS Compiler 6.2 : hdlDSPIP/DDS Compiler 6.0   partspresent=Phase_Generator_and_SIN_COS_LUT  dds_clock_rate=200  channels=1  mode_of_operation=Standard  output_type=Integer  modulus=9  parameter_entry=Hardware_Parameters  spurious_free_dynamic_range=45  frequency_resolution=0.4  noise_shaping=None  phase_width=24  output_width=16  output_selection=Sine_and_Cosine  negative_sine=off  negative_cosine=off  amplitude_mode=Full_Range  memory_type=Auto  optimization_goal=Auto  dsp48_use=Minimal  resync=off  latency_configuration=Auto  latency=1  has_phase_out=on  has_aclken=off  has_aresetn=off  explicit_period=on  period=1/200e6  data_has_tlast=Not_Required  has_tready=on  s_phase_has_tuser=Not_Required  m_data_has_tuser=Not_Required  m_phase_has_tuser=Not_Required  s_phase_tuser_width=1  output_form=Twos_Complement  s_config_sync_mode=On_Vector  phase_increment=Streaming  output_frequency1=0  output_frequency2=0  output_frequency3=0  output_frequency4=0  output_frequency5=0  output_frequency6=0  output_frequency7=0  output_frequency8=0  output_frequency9=0  output_frequency10=0  output_frequency11=0  output_frequency12=0  output_frequency13=0  output_frequency14=0  output_frequency15=0  output_frequency16=0  pinc1='0'  pinc2='0'  pinc3='0'  pinc4='0'  pinc5='0'  pinc6='0'  pinc7='0'  pinc8='0'  pinc9='0'  pinc10='0'  pinc11='0'  pinc12='0'  pinc13='0'  pinc14='0'  pinc15='0'  pinc16='0'  phase_offset=None  phase_offset_angles1=0  phase_offset_angles2=0  phase_offset_angles3=0  phase_offset_angles4=0  phase_offset_angles5=0  phase_offset_angles6=0  phase_offset_angles7=0  phase_offset_angles8=0  phase_offset_angles9=0  phase_offset_angles10=0  phase_offset_angles11=0  phase_offset_angles12=0  phase_offset_angles13=0  phase_offset_angles14=0  phase_offset_angles15=0  phase_offset_angles16=0  poff1='0'  poff2='0'  poff3='0'  poff4='0'  poff5='0'  poff6='0'  poff7='0'  poff8='0'  poff9='0'  poff10='0'  poff11='0'  poff12='0'  poff13='0'  poff14='0'  poff15='0'  poff16='0'  trim_axipin_name=on  simulation_type=hybrid_sim  simulation_model=sysgen:xddsv6_0_cmodel  data_path_portlist={ 's_axis_config_tdata_poff', 's_axis_config_tdata_chan0_poff', 's_axis_config_tdata_pinc', 's_axis_config_tdata_chan0_pinc', 's_axis_phase_tdata_resync', 's_axis_phase_tdata_chan0_resync', 's_axis_phase_tdata_poff', 's_axis_phase_tdata_chan0_poff', 's_axis_phase_tdata_pinc', 's_axis_phase_tdata_chan0_pinc', 's_axis_phase_tdata_phase_in', 'm_axis_data_tdata_sine', 'm_axis_data_tdata_chan0_sine', 'm_axis_data_tdata_cosine', 'm_axis_data_tdata_chan0_cosine', 'm_axis_phase_tdata_phase_out', 'm_axis_phase_tdata_chan0_phase_out'}  por_mode=false  gui_behaviour=Sysgen  ip_name=DDS Compiler  ip_version=6.0  dsptool_ready=true  wrapper_available=true  port_translation_map={ 'aclken' => 'en', 'aresetn' => 'rst' }  ipcore_usecache=true  ipcore_useipmodelcache=true  ipcore_xco_need_fpga_part=true  ipcore_fpga_part=[]  ipcore_verbose=false  XmcBlockStatus=1  maskContainerNames=tabcontainer1  block_type=dds_compiler_v6_0  block_config=sysgen:rodinimport_config  block_width=760
  DDS_Ready : hdlBasic/Constant  const=1  gui_display_data_type=Boolean  arith_type=Boolean  n_bits=24  bin_pt=0  preci_type=Single  exp_width=8  frac_width=24  explicit_period=on  period=1/200e6  XmcBlockStatus=1  maskContainerNames=tabcontainer1  block_type=constant  block_config=sysgen:Constant_config
  DebounceTmr : hdlBasic/Counter  cnt_type=Count limited  cnt_to=Btn_Debounce-1  operation=Up  start_count=0  cnt_by_val=1  arith_type=Unsigned  n_bits=18  bin_pt=0  load_pin=off  rst=on  en=on  explicit_period=Explicit  period=1/200e6  use_behavioral_HDL=off  implementation=Fabric  XmcBlockStatus=1  maskContainerNames=group1  block_type=counter  block_config=sysgen:Counter_config  block_width=531  block_height=1023
  DebounceTmr1 : hdlBasic/Counter  cnt_type=Count limited  cnt_to=Btn_Debounce-1  operation=Up  start_count=0  cnt_by_val=1  arith_type=Unsigned  n_bits=18  bin_pt=0  load_pin=off  rst=on  en=on  explicit_period=Explicit  period=1/200e6  use_behavioral_HDL=off  implementation=Fabric  XmcBlockStatus=1  maskContainerNames=group1  block_type=counter  block_config=sysgen:Counter_config  block_width=531  block_height=1023
  DebounceTmr2 : hdlBasic/Counter  cnt_type=Count limited  cnt_to=Btn_Debounce-1  operation=Up  start_count=0  cnt_by_val=1  arith_type=Unsigned  n_bits=18  bin_pt=0  load_pin=off  rst=on  en=on  explicit_period=Explicit  period=1/200e6  use_behavioral_HDL=off  implementation=Fabric  XmcBlockStatus=1  maskContainerNames=group1  block_type=counter  block_config=sysgen:Counter_config  block_width=531  block_height=1023
  DebounceTrig : hdlBasic/Relational  mode=a=b  op_type=Bool  en=off  latency=1  XmcBlockStatus=1  maskContainerNames=tabcontainer1  block_type=relational  block_config=sysgen:Relational_config
  DebounceTrig1 : hdlBasic/Relational  mode=a=b  op_type=Bool  en=off  latency=1  XmcBlockStatus=1  maskContainerNames=tabcontainer1  block_type=relational  block_config=sysgen:Relational_config
  DebounceTrig2 : hdlBasic/Relational  mode=a=b  op_type=Bool  en=off  latency=1  XmcBlockStatus=1  maskContainerNames=tabcontainer1  block_type=relational  block_config=sysgen:Relational_config
  Delay : hdlBasic/Delay  rst=off  en=off  latency=1  reg_retiming=off  XmcBlockStatus=1  maskContainerNames=group1  block_type=delay  block_config=sysgen:Delay_config
  DelayCM : hdlBasic/Delay  rst=off  en=off  latency=2  reg_retiming=off  XmcBlockStatus=1  maskContainerNames=group1  block_type=delay  block_config=sysgen:Delay_config
  FreqDeltaPeriod : hdlBasic/Constant  const=FreqDeltaPeriod  gui_display_data_type=Fixed-point  arith_type=Unsigned  n_bits=8  bin_pt=0  preci_type=Single  exp_width=8  frac_width=24  explicit_period=off  period=1  XmcBlockStatus=1  maskContainerNames=tabcontainer1  block_type=constant  block_config=sysgen:Constant_config
  FreqROMIncrementer : hdlBasic/Counter  cnt_type=Count limited  cnt_to=36  operation=Up  start_count=0  cnt_by_val=1  arith_type=Unsigned  n_bits=6  bin_pt=0  load_pin=off  rst=off  en=on  explicit_period=Inferred from inputs  period=1/100  use_behavioral_HDL=off  implementation=Fabric  XmcBlockStatus=1  maskContainerNames=group1  block_type=counter  block_config=sysgen:Counter_config  block_width=531  block_height=1023
  FreqRomSize : hdlBasic/Constant  const=36  gui_display_data_type=Fixed-point  arith_type=Unsigned  n_bits=8  bin_pt=0  preci_type=Single  exp_width=8  frac_width=24  explicit_period=off  period=1  XmcBlockStatus=1  maskContainerNames=tabcontainer1  block_type=constant  block_config=sysgen:Constant_config
  FrequencyROM : hdlBasic/ROM  depth=37  initVector=FCW  distributed_mem=Block RAM  rst=off  init_reg=0  en=off  latency=1  gui_display_data_type=Fixed-point  arith_type=Unsigned  n_bits=24  bin_pt=24  preci_type=Double  exp_width=8  frac_width=24  optimize=Area  use_rpm=on  simulation_type=fast_sim  XmcBlockStatus=1  maskContainerNames=tabcontainer1  block_type=sprom  block_config=sysgen:SPROM_config
  FrequencyShiftROM : hdlBasic/ROM  depth=9  initVector=DPShift_Rom  distributed_mem=Block RAM  rst=off  init_reg=0  en=off  latency=1  gui_display_data_type=Fixed-point  arith_type=Unsigned  n_bits=24  bin_pt=24  preci_type=Double  exp_width=8  frac_width=24  optimize=Area  use_rpm=on  simulation_type=fast_sim  XmcBlockStatus=1  maskContainerNames=tabcontainer1  block_type=sprom  block_config=sysgen:SPROM_config
  Mux : hdlBasic/Mux  inputs=2  en=off  latency=0  precision=Full  arith_type=Unsigned  n_bits=16  bin_pt=14  quantization=Truncate  overflow=Wrap  XmcBlockStatus=1  maskContainerNames=tabcontainer1  block_type=mux  block_config=sysgen:Mux_config
  PhaseROM : hdlBasic/ROM  depth=11  initVector=phi_norm  distributed_mem=Block RAM  rst=off  init_reg=0  en=off  latency=1  gui_display_data_type=Fixed-point  arith_type=Unsigned  n_bits=24  bin_pt=24  preci_type=Double  exp_width=8  frac_width=24  optimize=Area  use_rpm=on  simulation_type=fast_sim  XmcBlockStatus=1  maskContainerNames=tabcontainer1  block_type=sprom  block_config=sysgen:SPROM_config
  ROM : hdlBasic/ROM  depth=2  initVector=[0,1]  distributed_mem=Block RAM  rst=off  init_reg=0  en=off  latency=1  gui_display_data_type=Boolean  arith_type=Boolean  n_bits=16  bin_pt=14  preci_type=Single  exp_width=8  frac_width=24  optimize=Area  use_rpm=on  simulation_type=fast_sim  XmcBlockStatus=1  maskContainerNames=tabcontainer1  block_type=sprom  block_config=sysgen:SPROM_config
  RstHold1 : hdlBasic/Inverter  en=off  latency=0  XmcBlockStatus=1  maskContainerNames=group2  block_type=inv  block_config=sysgen:Inverter_config
  RstHold2 : hdlBasic/Inverter  en=off  latency=0  XmcBlockStatus=1  maskContainerNames=group2  block_type=inv  block_config=sysgen:Inverter_config
  RstHold3 : hdlBasic/Inverter  en=off  latency=0  XmcBlockStatus=1  maskContainerNames=group2  block_type=inv  block_config=sysgen:Inverter_config
  SweepCRelational : hdlBasic/Relational  mode=a=b  op_type=Bool  en=off  latency=0  XmcBlockStatus=1  maskContainerNames=tabcontainer1  block_type=relational  block_config=sysgen:Relational_config
  SweepCounter : hdlBasic/Counter  cnt_type=Count limited  cnt_to=SweepTime-1  operation=Up  start_count=0  cnt_by_val=1  arith_type=Unsigned  n_bits=32  bin_pt=0  load_pin=off  rst=off  en=off  explicit_period=Explicit  period=1/200e6  use_behavioral_HDL=off  implementation=Fabric  XmcBlockStatus=1  maskContainerNames=group1  block_type=counter  block_config=sysgen:Counter_config  block_width=531  block_height=1023
  SweepTime : hdlBasic/Constant  const=SweepTime-1  gui_display_data_type=Fixed-point  arith_type=Unsigned  n_bits=24  bin_pt=0  preci_type=Single  exp_width=8  frac_width=24  explicit_period=off  period=1  XmcBlockStatus=1  maskContainerNames=tabcontainer1  block_type=constant  block_config=sysgen:Constant_config
  Terminator{,1..13} (14 alike) : Terminator
  TimeHoldTrig : hdlBasic/Constant  const=Btn_Debounce-1  gui_display_data_type=Fixed-point  arith_type=Unsigned  n_bits=18  bin_pt=0  preci_type=Single  exp_width=8  frac_width=24  explicit_period=off  period=1  XmcBlockStatus=1  maskContainerNames=tabcontainer1  block_type=constant  block_config=sysgen:Constant_config
  TimeHoldTrig1 : hdlBasic/Constant  const=Btn_Debounce-1  gui_display_data_type=Fixed-point  arith_type=Unsigned  n_bits=18  bin_pt=0  preci_type=Single  exp_width=8  frac_width=24  explicit_period=off  period=1  XmcBlockStatus=1  maskContainerNames=tabcontainer1  block_type=constant  block_config=sysgen:Constant_config
  TimeHoldTrig2 : hdlBasic/Constant  const=Btn_Debounce-1  gui_display_data_type=Fixed-point  arith_type=Unsigned  n_bits=18  bin_pt=0  preci_type=Single  exp_width=8  frac_width=24  explicit_period=off  period=1  XmcBlockStatus=1  maskContainerNames=tabcontainer1  block_type=constant  block_config=sysgen:Constant_config
  Out7 : Outport
  Out8 : Outport  Port=2
  Out10 : Outport  Port=3
  Out6 : Outport  Port=4
  Out2 : Outport  Port=5
  Out3 : Outport  Port=6
  Out5 : Outport  Port=7
  Out4 : Outport  Port=8
  Out1 : Outport  Port=9
  Out9 : Outport  Port=10
  Out11 : Outport  Port=11
  wires:
  ChirpCounter/1 -> ChirpCRelational/1
  In9/1 -> Button In2/1
  Button In3/1 -> RstHold1/1, DebounceTmr/2
  DDS Compiler 6.1/3 -> Out5/1, Mux/2, CMult/1  "TX2SrcQ"
  Mux/1 -> Addressable Shift Register3/1
  DDS Compiler 6.0/3 -> Out2/1, Addressable Shift Register1/1  "TX1SrcQ"
  DebounceTrig1/1 -> Counter1/1
  FrequencyROM/1 -> DDS Compiler 6.1/2, DDS Compiler 6.0/3
  CMult/1 -> Mux/3
  DebounceTmr/1 -> DebounceTrig/1
  ChirpCRelational/1 -> Out1/1, FreqROMIncrementer/1  "ChirpTrigger"
  PhaseROM/1 -> DDS Compiler 6.0/2
  FreqDeltaPeriod/1 -> ChirpCRelational/2
  Addressable Shift Register3/1 -> Complex Multiplier 6.1/2
  Delay/1 -> DDS Compiler 6.1/4, DDS Compiler 6.1/3, DDS Compiler 6.1/1, DDS Compiler 6.2/4, DDS Compiler 6.2/3, DDS Compiler 6.2/1, DDS Compiler 6.0/5, DDS Compiler 6.0/4, DDS Compiler 6.0/1
  DebounceTrig/1 -> BtnIncrementPhasor/1
  CM_Ready/1 -> DelayCM/1
  TimeHoldTrig/1 -> DebounceTrig/2
  DDS Compiler 6.2/4 -> Complex Multiplier 6.0/6, Complex Multiplier 6.1/6
  SweepCounter/1 -> SweepCRelational/1
  Complex Multiplier 6.1/3 -> Out6/1  "TX2I"
  AngleCounter/1 -> AngleCRelational/1
  TimeHoldTrig1/1 -> DebounceTrig1/2
  AngleIncrementer/1 -> PhaseROM/1
  DDS_Ready/1 -> Delay/1
  Addressable Shift Register2/1 -> Convert/1
  In2/1 -> Button In3/1
  Complex Multiplier 6.1/2 -> Out10/1  "TX2Q"
  BtnIncrementPhasor/1 -> FrequencyShiftROM/1
  Button In1/1 -> RstHold2/1, DebounceTmr1/2
  SweepTime/1 -> SweepCRelational/2
  RstHold1/1 -> DebounceTmr/1
  AngleTime/1 -> AngleCRelational/2
  Counter1/1 -> Addressable Shift Register2/2, Addressable Shift Register3/2, Addressable Shift Register1/2, Addressable Shift Register/2
  FreqROMIncrementer/1 -> ChirpPeriodRel/1, FrequencyROM/1
  DDS Compiler 6.1/4 -> Out4/1, Addressable Shift Register2/1  "TX2SrcI"
  DebounceTmr2/1 -> DebounceTrig2/1
  In1/1 -> Button In1/1
  Convert/1 -> Complex Multiplier 6.1/3
  FrequencyShiftROM/1 -> DDS Compiler 6.2/2
  TimeHoldTrig2/1 -> DebounceTrig2/2
  DDS Compiler 6.2/3 -> Complex Multiplier 6.1/5, Complex Multiplier 6.0/5
  Complex Multiplier 6.0/2 -> Out7/1  "TX1Q"
  RstHold3/1 -> DebounceTmr2/1
  Counter2/1 -> ROM/1
  Addressable Shift Register1/1 -> Complex Multiplier 6.0/2
  DDS Compiler 6.0/6 -> Terminator/1
  Complex Multiplier 6.1/1 -> Terminator12/1
  Complex Multiplier 6.0/3 -> Out8/1  "TX1I"
  DebounceTmr1/1 -> DebounceTrig1/1
  DebounceTrig2/1 -> Counter2/1
  ROM/1 -> Mux/1
  DelayCM/1 -> Complex Multiplier 6.1/4, Complex Multiplier 6.1/1, Complex Multiplier 6.0/4, Complex Multiplier 6.0/1
  Button In2/1 -> RstHold3/1, DebounceTmr2/2
  RstHold2/1 -> DebounceTmr1/1
  Addressable Shift Register/1 -> Complex Multiplier 6.0/3
  DDS Compiler 6.0/4 -> Out3/1, Addressable Shift Register/1  "TX1SrcI"
  DDS Compiler 6.0/2 -> Terminator2/1  "Signl"
  DDS Compiler 6.1/1 -> Terminator11/1
  DDS Compiler 6.0/5 -> Terminator1/1
  DDS Compiler 6.1/2 -> Terminator10/1
  DDS Compiler 6.2/1 -> Terminator7/1
  DDS Compiler 6.1/5 -> Terminator9/1
  Complex Multiplier 6.0/1 -> Terminator13/1
  DDS Compiler 6.1/6 -> Terminator8/1
  DDS Compiler 6.2/6 -> Terminator4/1
  DDS Compiler 6.0/1 -> Terminator3/1
  DDS Compiler 6.2/2 -> Terminator6/1  "Signl"
  DDS Compiler 6.2/5 -> Terminator5/1
  AngleCRelational/1 -> Out9/1, AngleIncrementer/2  "FrameToggle"
  SweepCRelational/1 -> AngleIncrementer/1
  FreqRomSize/1 -> ChirpPeriodRel/2
  ChirpPeriodRel/1 -> Out11/1  "ChirpPeriod"
